simulink model "sampleModel1970"  (R2023a)
settings: Solver=VariableStepAuto  StartTime=0.0  StopTime=10.0  RelTol=1e-3
libraries: hdlsllib x8, simulink x4
settings Model: Creator=user1  LastModifiedBy=user1

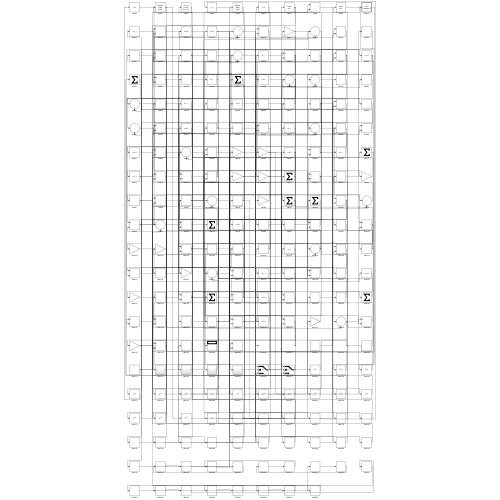
[thumbnail: Simulink's stored preview of the top-level diagram]
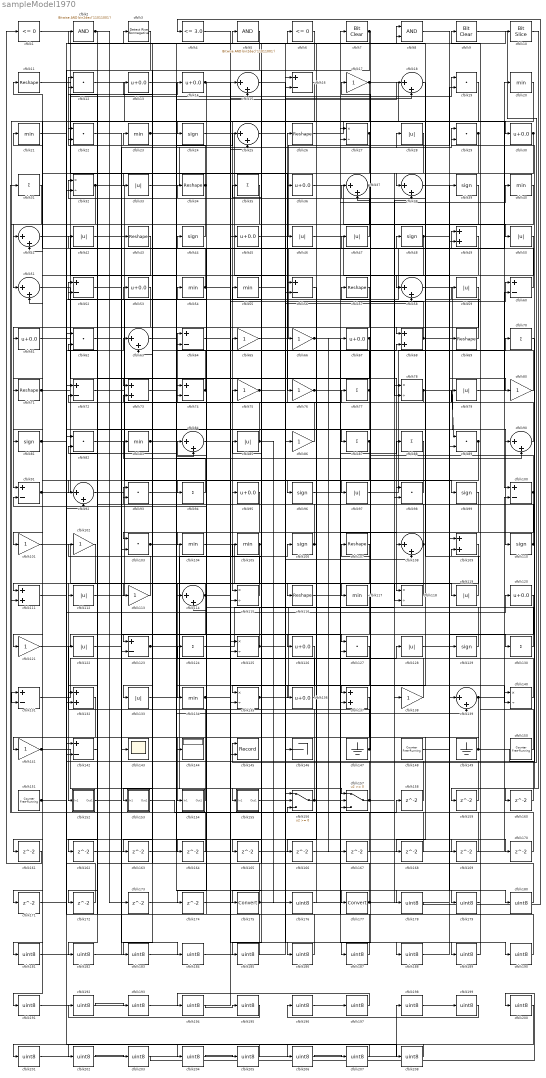
== system sampleModel1970 ==
  cfblk1 : hdlsllib/Logic and Bit Operations/Compare To Zero  relop=<=  OutDataTypeStr=boolean
  cfblk10 : hdlsllib/Logic and Bit Operations/Bit Slice  lidx=7  ridx=0
  cfblk{16,52,56,60,64,72,74,91,100,123,131,142} (12 alike) : Sum  Inputs=+-
  cfblk{17,65..66,75..76,80,86,101..102,113,121,138,141} (13 alike) : Gain
  cfblk{12,19,22,29,62,82,89,93,98,103,127} (11 alike) : DotProduct  OutDataTypeStr=Inherit: Inherit via internal rule
  cfblk{20..21,23,40,54..55,83,104..105,117,134} (11 alike) : MinMax
  cfblk{24,39,44,48,81,96,99,106,110,129} (10 alike) : Signum
  cfblk{11,26,34,43,57,69,71,107,116} (9 alike) : Reshape
  cfblk{15,18,25,37..38,41,51,58,63,84,90,92,108,114,139} (15 alike) : Sum  Inputs=|++
  cfblk{49,68,73,109,111,132,137} (7 alike) : Sum
  cfblk{28,33,42,46..47,50,59,79,85,97,112,119,122,128,133} (15 alike) : Abs  SaturateOnIntegerOverflow=off
  cfblk{27,32,78,115,118,125,135,140} (8 alike) : Product  Inputs=*/  RndMeth=Zero  SaturateOnIntegerOverflow=on
  cfblk{13..14,30,36,45,53,61,67,95,120,126,136} (12 alike) : Bias  Bias=0.0  SaturateOnIntegerOverflow=off
  cfblk{31,35,70,77,87..88,94,124,130} (9 alike) : Sum  Inputs=+
  cfblk143 : Scope
  cfblk144 : Display
  cfblk145 : Record  FileSettingsInternal="{\"entries\":[{\"content\":{\"excelSettings\":{\"content\":{},\"type\":\"Streamout.ExcelSettings\"}},\"type\":\"Streamout.FileSettingStorage\",\"uuid\":\"\"}],\"packageUris\":[\"http:\\/\\/schema.mathworks.com\\/mf0\\/streamout_blocks\\/R2020a\"],\"version\":\"1.0\"}"  Layout=[1 1]  SignalsInternal="{\"entries\":[{\"content\":{\"signals\":[{\"content\":{\"blockPath\":[],\"dimensions\":[1],\"domain\":\"\",\"lineColor\":\"#a2142f\",\"plots\":[1],\"port\":1,\"signalID\":5563,\"signalName\":\"XY Graph:1\"},\"type\":\"RecordBlkView.Signal\",\"uuid\":\"\"},{\"content\":{\"blockPath\":[],\"dimensions\":[1],\"domain\":\"\",\"lineColor\":\"#139fff\",\"plots\":[1],\"port\":2,\"signalID\":5566,\"signalName\":\"XY Graph:2\"},\"type\":\"RecordBlkView.Signal\",\"uuid\":\"\"}]},\"type\":\"RecordBlkView.InputSignals\",\"uuid\":\"\"}],\"packageUris\":[\"http:\\/\\/schema.mathworks.com\\/mf0\\/streamout_blocks\\/R2020a\"],\"version\":\"1.0\"}"  VisualizationBindings="{\"xyplotplugin\":{\"info\":[{\"series\":[{\"bindingParametersList\":[{\"parameter\":\"X-Axis\",\"signalID\":5563,\"signalName\":\"XY Graph:1\"},{\"parameter\":\"Y-Axis\",\"signalID\":5566,\"signalName\":\"XY Graph:2\"}],\"seriesID\":15514}],\"subplotID\":1}]}}"  CompatibilityTag=XY  st=-1
  cfblk146 : Terminator
  cfblk147 : Ground
  cfblk148 : hdlsllib/Sources/Counter Free-Running  NumBits=16  tsamp=-1
  cfblk149 : Ground
  cfblk150 : hdlsllib/Sources/Counter Free-Running  NumBits=16  tsamp=-1
  cfblk151 : hdlsllib/Sources/Counter Free-Running  NumBits=16  tsamp=-1
  cfblk152 : Subsystem
      settings: LibrarySourceBlock=|
      | hdlsllib/Ports &
      | Subsystems/Subsystem
  cfblk153 : Subsystem
      settings: LibrarySourceBlock=|
      | hdlsllib/Ports &
      | Subsystems/Subsystem
  cfblk154 : Subsystem
      settings: LibrarySourceBlock=|
      | hdlsllib/Ports &
      | Subsystems/Subsystem
  cfblk155 : Subsystem
      settings: LibrarySourceBlock=|
      | hdlsllib/Ports &
      | Subsystems/Subsystem
  cfblk156 : Switch  SaturateOnIntegerOverflow=off  InputSameDT=off
  cfblk157 : Switch  SaturateOnIntegerOverflow=off  InputSameDT=off
  cfblk{158..174} (17 alike) : Delay  SampleTime=1
  cfblk175 : DataTypeConversion  SaturateOnIntegerOverflow=off  RndMeth=Floor
  cfblk{176,178..208} (32 alike) : DataTypeConversion  OutDataTypeStr=uint8  SaturateOnIntegerOverflow=off  RndMeth=Floor
  cfblk177 : DataTypeConversion  SaturateOnIntegerOverflow=off  RndMeth=Floor
  cfblk2 : simulink/Logic and Bit Operations/Bitwise Operator  logicop=AND  UseBitMask=on  BitMask=bin2dec('11011001')  BitMaskRealWorld=Stored Integer
      settings: LibrarySourceBlock=|
      | hdlsllib/Logic and Bit
      | Operations/Bitwise
      | Operator
  cfblk3 : hdlsllib/Logic and Bit Operations/Detect Rise Nonnegative  vinit=0  OutDataTypeStr=boolean
  cfblk4 : hdlsllib/Logic and Bit Operations/Compare To Constant  relop=<=  const=3.0  OutDataTypeStr=boolean
  cfblk5 : simulink/Logic and Bit Operations/Bitwise Operator  logicop=AND  UseBitMask=on  BitMask=bin2dec('11011001')  BitMaskRealWorld=Stored Integer
      settings: LibrarySourceBlock=|
      | hdlsllib/Logic and Bit
      | Operations/Bitwise
      | Operator
  cfblk6 : hdlsllib/Logic and Bit Operations/Compare To Zero  relop=<=  OutDataTypeStr=boolean
  cfblk7 : simulink/Logic and Bit Operations/Bit Clear  iBit=0
      settings: LibrarySourceBlock=|
      | hdlsllib/Logic and Bit
      | Operations/Bit Clear
  cfblk8 : Logic  AllPortsSameDT=off  OutDataTypeStr=boolean
  cfblk9 : simulink/Logic and Bit Operations/Bit Clear  iBit=0
      settings: LibrarySourceBlock=|
      | hdlsllib/Logic and Bit
      | Operations/Bit Clear
  wires:
  cfblk98/1 -> cfblk94/1
  cfblk91/1 -> cfblk48/1, cfblk18/1
  cfblk92/1 -> cfblk77/1
  cfblk11/1 -> cfblk24/1
  cfblk105/1 -> cfblk152/1(In1), cfblk35/1
  cfblk72/1 -> cfblk54/1
  cfblk40/1 -> cfblk135/1
  cfblk138/1 -> cfblk57/1
  cfblk26/1 -> cfblk30/1
  cfblk118/1 -> cfblk112/1
  cfblk31/1 -> cfblk51/1
  cfblk53/1 -> cfblk91/1
  cfblk19/1 -> cfblk115/1
  cfblk71/1 -> cfblk19/1, cfblk56/1
  cfblk85/1 -> cfblk64/1, cfblk176/1
  cfblk150/1 -> cfblk64/2
  cfblk2/1 -> cfblk172/1, cfblk173/1
  cfblk149/1 -> cfblk29/1, cfblk141/1
  cfblk59/1 -> cfblk61/1
  cfblk119/1 -> cfblk3/1
  cfblk142/1 -> cfblk31/1
  cfblk108/1 -> cfblk44/1, cfblk126/1, cfblk22/2
  cfblk61/1 -> cfblk14/1
  cfblk121/1 -> cfblk123/1
  cfblk30/1 -> cfblk117/1, cfblk121/1
  cfblk130/1 -> cfblk84/1
  cfblk32/1 -> cfblk97/1, cfblk111/2
  cfblk29/1 -> cfblk38/1, cfblk78/2
  cfblk9/1 -> cfblk145/1
  cfblk51/1 -> cfblk118/1
  cfblk69/1 -> cfblk32/1
  cfblk111/1 -> cfblk10/1
  cfblk4/1 -> cfblk177/1
  cfblk97/1 -> cfblk70/1
  cfblk86/1 -> cfblk26/1
  cfblk133/1 -> cfblk106/1
  cfblk43/1 -> cfblk71/1
  cfblk38/1 -> cfblk129/1
  cfblk39/1 -> cfblk51/2
  cfblk1/1 -> cfblk76/1
  cfblk83/1 -> cfblk65/1, cfblk75/1, cfblk8/1
  cfblk42/1 -> cfblk87/1
  cfblk122/1 -> cfblk29/2
  cfblk57/1 -> cfblk81/1
  cfblk67/1 -> cfblk145/2, cfblk92/1
  cfblk78/1 -> cfblk89/1, cfblk73/2
  cfblk112/1 -> cfblk20/1
  cfblk81/1 -> cfblk89/2, cfblk208/1
  cfblk54/1 -> cfblk11/1, cfblk99/1
  cfblk120/1 -> cfblk123/2
  cfblk90/1 -> cfblk5/1
  cfblk36/1 -> cfblk50/1
  cfblk52/1 -> cfblk116/1
  cfblk135/1 -> cfblk67/1, cfblk18/2
  cfblk88/1 -> cfblk135/2
  cfblk103/1 -> cfblk157/1, cfblk25/1
  cfblk107/1 -> cfblk115/2
  cfblk24/1 -> cfblk86/1
  cfblk131/1 -> cfblk128/1
  cfblk75/1 -> cfblk49/1, cfblk58/2
  cfblk58/1 -> cfblk110/1
  cfblk56/1 -> cfblk136/1
  cfblk87/1 -> cfblk96/1, cfblk101/1
  cfblk148/1 -> cfblk39/1
  cfblk101/1 -> cfblk134/1
  cfblk46/1 -> cfblk139/1
  cfblk137/1 -> cfblk154/1(In1)
  cfblk124/1 -> cfblk78/1
  cfblk68/1 -> cfblk17/1, cfblk130/1
  cfblk63/1 -> cfblk84/2
  cfblk156/1 -> cfblk122/1, cfblk40/1, cfblk88/1
  cfblk64/1 -> cfblk90/1
  cfblk116/1 -> cfblk7/1
  cfblk34/1 -> cfblk12/1, cfblk41/2
  cfblk20/1 -> cfblk98/1
  cfblk76/1 -> cfblk27/2, cfblk118/2
  cfblk14/1 -> cfblk127/2, cfblk25/2, cfblk174/1
  cfblk89/1 -> cfblk95/1, cfblk171/1
  cfblk33/1 -> cfblk28/1
  cfblk134/1 -> cfblk60/1, cfblk68/2
  cfblk93/1 -> cfblk139/2
  cfblk17/1 -> cfblk100/1, cfblk131/2
  cfblk141/1 -> cfblk155/1(In1), cfblk92/2
  cfblk140/1 -> cfblk74/2
  cfblk74/1 -> cfblk23/1, cfblk22/1
  cfblk60/1 -> cfblk21/1
  cfblk114/1 -> cfblk153/1(In1), cfblk111/1, cfblk140/2
  cfblk132/1 -> cfblk142/2
  cfblk110/1 -> cfblk93/1, cfblk79/1
  cfblk7/1 -> cfblk32/2, cfblk37/2
  cfblk154/1(Out1) -> cfblk52/1
  cfblk5/1 -> cfblk33/1
  cfblk45/1 -> cfblk19/2
  cfblk82/1 -> cfblk114/1
  cfblk104/1 -> cfblk146/1
  cfblk129/1 -> cfblk91/2
  cfblk6/1 -> cfblk175/1
  cfblk27/1 -> cfblk36/1, cfblk103/2, cfblk183/1
  cfblk79/1 -> cfblk60/2
  cfblk151/1 -> cfblk63/1, cfblk120/1
  cfblk106/1 -> cfblk63/2, cfblk66/1
  cfblk65/1 -> cfblk47/1
  cfblk37/1 -> cfblk56/2, cfblk185/1
  cfblk12/1 -> cfblk69/1
  cfblk3/1 -> cfblk132/1
  cfblk100/1 -> cfblk37/1, cfblk133/1, cfblk164/1
  cfblk115/1 -> cfblk102/1
  cfblk23/1 -> cfblk119/1, cfblk73/1
  cfblk139/1 -> cfblk100/2, cfblk168/1
  cfblk44/1 -> cfblk41/1
  cfblk41/1 -> cfblk144/1
  cfblk123/1 -> cfblk156/1, cfblk90/2
  cfblk66/1 -> cfblk108/1, cfblk167/1
  cfblk22/1 -> cfblk127/1
  cfblk48/1 -> cfblk58/1, cfblk80/1
  cfblk80/1 -> cfblk9/1
  cfblk77/1 -> cfblk2/1, cfblk182/1
  cfblk99/1 -> cfblk103/1
  cfblk25/1 -> cfblk108/2
  cfblk157/1 -> cfblk38/2, cfblk46/1
  cfblk47/1 -> cfblk34/1
  cfblk152/1(Out1) -> cfblk143/1
  cfblk50/1 -> cfblk113/1
  cfblk147/1 -> cfblk107/1, cfblk85/1
  cfblk136/1 -> cfblk105/1
  cfblk94/1 -> cfblk83/1
  cfblk18/1 -> cfblk68/1
  cfblk95/1 -> cfblk104/1
  cfblk113/1 -> cfblk82/2
  cfblk125/1 -> cfblk52/2, cfblk72/2, cfblk8/2
  cfblk73/1 -> cfblk137/1
  cfblk49/1 -> cfblk125/2
  cfblk153/1(Out1) -> cfblk158/1
  cfblk158/1 -> cfblk27/1
  cfblk10/1 -> cfblk159/1
  cfblk159/1 -> cfblk82/1
  cfblk70/1 -> cfblk160/1
  cfblk160/1 -> cfblk12/2
  cfblk102/1 -> cfblk161/1
  cfblk161/1 -> cfblk1/1
  cfblk35/1 -> cfblk162/1
  cfblk162/1 -> cfblk125/1
  cfblk117/1 -> cfblk163/1
  cfblk163/1 -> cfblk74/1
  cfblk164/1 -> cfblk93/2
  cfblk126/1 -> cfblk165/1
  cfblk165/1 -> cfblk98/2
  cfblk127/1 -> cfblk166/1
  cfblk166/1 -> cfblk140/1
  cfblk167/1 -> cfblk114/2
  cfblk168/1 -> cfblk156/3
  cfblk21/1 -> cfblk169/1
  cfblk169/1 -> cfblk142/1
  cfblk128/1 -> cfblk170/1
  cfblk170/1 -> cfblk131/1
  cfblk171/1 -> cfblk132/2
  cfblk172/1 -> cfblk72/1
  cfblk173/1 -> cfblk156/2
  cfblk174/1 -> cfblk49/2
  cfblk175/1 -> cfblk137/2, cfblk13/1, cfblk157/3, cfblk138/1
  cfblk176/1 -> cfblk6/1
  cfblk177/1 -> cfblk42/1, cfblk53/1
  cfblk13/1 -> cfblk178/1
  cfblk178/1 -> cfblk4/1
  cfblk55/1 -> cfblk179/1
  cfblk179/1 -> cfblk59/1
  cfblk8/1 -> cfblk180/1
  cfblk180/1 -> cfblk55/1
  cfblk16/1 -> cfblk181/1
  cfblk181/1 -> cfblk43/1
  cfblk182/1 -> cfblk16/1
  cfblk183/1 -> cfblk16/2
  cfblk62/1 -> cfblk184/1
  cfblk184/1 -> cfblk45/1
  cfblk185/1 -> cfblk62/1
  cfblk84/1 -> cfblk186/1
  cfblk186/1 -> cfblk62/2
  cfblk109/1 -> cfblk187/1
  cfblk187/1 -> cfblk124/1
  cfblk96/1 -> cfblk188/1
  cfblk188/1 -> cfblk109/1
  cfblk155/1(Out1) -> cfblk189/1
  cfblk189/1 -> cfblk109/2
  cfblk15/1 -> cfblk190/1
  cfblk190/1 -> cfblk157/2
  cfblk28/1 -> cfblk191/1
  cfblk191/1 -> cfblk15/1
  cfblk192/1 -> cfblk193/1
  cfblk193/1 -> cfblk15/2
  cfblk194/1 -> cfblk195/1
  cfblk195/1 -> cfblk192/1
  cfblk196/1 -> cfblk197/1
  cfblk197/1 -> cfblk194/1
  cfblk198/1 -> cfblk199/1
  cfblk199/1 -> cfblk196/1
  cfblk200/1 -> cfblk201/1
  cfblk201/1 -> cfblk198/1
  cfblk202/1 -> cfblk203/1
  cfblk203/1 -> cfblk200/1
  cfblk204/1 -> cfblk205/1
  cfblk205/1 -> cfblk202/1
  cfblk206/1 -> cfblk207/1
  cfblk207/1 -> cfblk204/1
  cfblk208/1 -> cfblk206/1

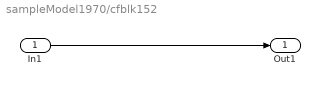
== system sampleModel1970/cfblk152 ==
  In1 : Inport
  Out1 : Outport
  wires:
  In1/1 -> Out1/1

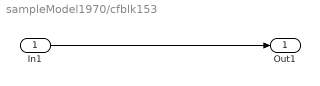
== system sampleModel1970/cfblk153 ==
  In1 : Inport
  Out1 : Outport
  wires:
  In1/1 -> Out1/1

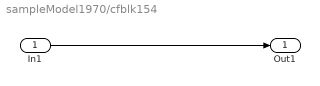
== system sampleModel1970/cfblk154 ==
  In1 : Inport
  Out1 : Outport
  wires:
  In1/1 -> Out1/1

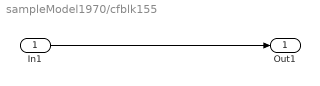
== system sampleModel1970/cfblk155 ==
  In1 : Inport
  Out1 : Outport
  wires:
  In1/1 -> Out1/1
